simulink model "attitude_cbf"  (R2020b)
settings: Solver=VariableStepAuto  StartTime=0.0  StopTime=10.0  RelTol=1e-3
settings Model: Creator=kt012  LastModifiedBy=kt012

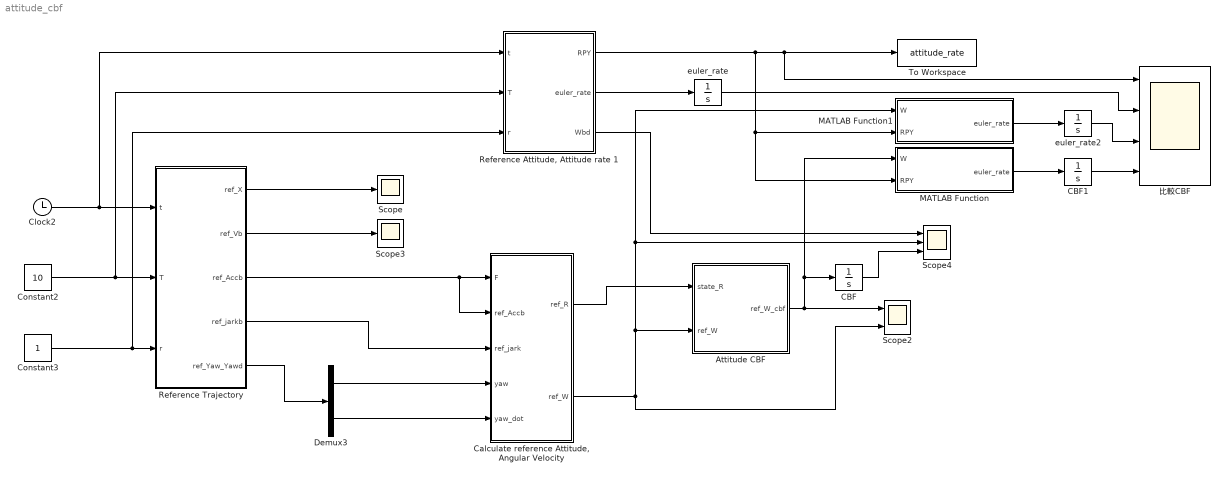
== system attitude_cbf ==
  Attitude CBF : MATLAB Function  TreatAsAtomicUnit=on
  CBF : Integrator  InitialCondition=[0.0403 0 0];
  CBF1 : Integrator  InitialCondition=[0.0403 0 0];
  "Calculate reference Attitude, Angular Velocity" : MATLAB Function  TreatAsAtomicUnit=on
  Clock2 : Clock
  Constant2 : Constant  Value=10
  Constant3 : Constant
  Demux3 : Demux  Outputs=2
  MATLAB Function : MATLAB Function  TreatAsAtomicUnit=on
  MATLAB Function1 : MATLAB Function  TreatAsAtomicUnit=on
  "Reference Attitude, Attitude rate 1" : MATLAB Function  TreatAsAtomicUnit=on
  Reference Trajectory : MATLAB Function  TreatAsAtomicUnit=on
  Scope : Scope
  Scope2 : Scope  NumInputPorts=2
  Scope3 : Scope
  Scope4 : Scope  NumInputPorts=3
  To Workspace : ToWorkspace  VariableName=attitude_rate  SaveFormat=Structure  SampleTime=-1
  euler_rate : Integrator  InitialCondition=[0.0403 0 0];
  euler_rate2 : Integrator  InitialCondition=[0.0403 0 0];
  比較CBF : Scope  NumInputPorts=4
  wires:
  Clock2/1 -> "Reference Attitude, Attitude rate 1"/1(t), Reference Trajectory/1(t)
  Constant3/1 -> "Reference Attitude, Attitude rate 1"/3(r), Reference Trajectory/3(r)
  Constant2/1 -> "Reference Attitude, Attitude rate 1"/2(T), Reference Trajectory/2(T)
  Reference Trajectory/1(ref_X) -> Scope/1
  Reference Trajectory/2(ref_Vb) -> Scope3/1
  Reference Trajectory/3(ref_Accb) -> "Calculate reference Attitude, Angular Velocity"/2(ref_Accb), "Calculate reference Attitude, Angular Velocity"/1(F)
  Reference Trajectory/4(ref_jarkb) -> "Calculate reference Attitude, Angular Velocity"/3(ref_jark)
  Reference Trajectory/5(ref_Yaw_Yawd) -> Demux3/1
  Demux3/1 -> "Calculate reference Attitude, Angular Velocity"/4(yaw)
  Demux3/2 -> "Calculate reference Attitude, Angular Velocity"/5(yaw_dot)
  "Calculate reference Attitude, Angular Velocity"/1(ref_R) -> Attitude CBF/1(state_R)
  "Calculate reference Attitude, Angular Velocity"/2(ref_W) -> Scope2/2, MATLAB Function1/1(W), Scope4/2, Attitude CBF/2(ref_W)
  Attitude CBF/1(ref_W_cbf) -> Scope2/1, MATLAB Function/1(W), CBF/1
  "Reference Attitude, Attitude rate 1"/3(Wbd) -> Scope4/1
  "Reference Attitude, Attitude rate 1"/1(RPY) -> MATLAB Function/2(RPY), MATLAB Function1/2(RPY), 比較CBF/1, To Workspace/1
  CBF/1 -> Scope4/3
  "Reference Attitude, Attitude rate 1"/2(euler_rate) -> euler_rate/1
  euler_rate/1 -> 比較CBF/2
  euler_rate2/1 -> 比較CBF/3
  MATLAB Function/1(euler_rate) -> CBF1/1
  MATLAB Function1/1(euler_rate) -> euler_rate2/1
  CBF1/1 -> 比較CBF/4

== matlab function attitude_cbf/Reference Attitude, Attitude rate 1 ==
  data: RPY output; euler_rate output; Wbd output; t input; T input; r input
function [RPY, euler_rate, Wbd] = fcn(t,T,r)
% 軌道生成
w = 2 * pi/T;          % 角周波数

% 中心　半径　　
c = [0;0;0];

% Flat Outputから内部状態と入力揚力を計算
% 各軸の単位行列
e1 = [1; 0; 0];e2 = [0; 1; 0];e3 = [0; 0; 1];
% ドローンの質量　重力加速度
mQ = 0.027; g = 9.8;


x = c + r*[sin(w*t); cos(w*t); 0];         % 位置の軌道の位置
dx = r*[w*cos(w*t); -w*sin(w*t); 0];       % 速度の軌道
d2x = r*[-w^2*sin(w*t); -w^2*cos(w*t); 0]; % 加速度の軌道
d3x = r*[-w^3*cos(w*t); w^3*sin(w*t); 0];  % 加加速度の軌道
d4x = r*[w^4*sin(w*t); w^4*cos(w*t); 0];   % 加加加速度の軌道

alpha = 0;                                 
d_alpha = 0;                               
d2x(3) = d2x(3)+g;

pitch = atan( ( d2x(1)*cos(alpha) + d2x(2)*sin(alpha) ) / (d2x(3)));                                                        
roll = atan( ( d2x(1)*sin(alpha) - d2x(2)*cos(alpha) ) / sqrt( (d2x(3))^2 + ( d2x(1)*cos(alpha) + d2x(2)*sin(alpha) )^2));

rollS = sin(roll); rollC = cos(roll);           
pitchS = sin(pitch); pitchC = cos(pitch);       
yawS = sin(alpha); yawC = cos(alpha);           


% desired Roll rate
roll_rate_bunshi = d2x(3)^2 * ( d3x(1)*yawS - d3x(2)*yawC + d_alpha * (d2x(1)*yawC + d2x(2)*yawS) ) - d2x(3)*d3x(3)*(d2x(1)*yawS - d2x(2)*yawC) + (d2x(1)*yawC + d2x(2)*yawS)*(d_alpha*(d2x(1)^2 + d2x(2)^2) - d2x(1)*d3x(2) + d2x(2)*d3x(1));
roll_rate_bunbo = (d2x(1)^2 + d2x(2)^2 + d2x(3)^2) * sqrt(d2x(3)^2 + ( d2x(1)*yawC + d2x(2)*yawS )^2);
roll_rate = roll_rate_bunshi / roll_rate_bunbo;

% desired Pitch rate
pitch_rate_bunshi = d2x(3)*(d3x(1)*yawC + d3x(2)*yawS) - d3x(3)*(d2x(1)*yawC + d2x(2)*yawS) - d2x(3)*d_alpha*(d2x(1)*yawS + d2x(2)*yawC);
pitch_rate_bunbo = d2x(3)^2 + ( d2x(1)*yawC + d2x(2)*yawS )^2;
pitch_rate = pitch_rate_bunshi / pitch_rate_bunbo;

W = [1 0      -pitchS;
     0 rollC  pitchC * rollS;
     0 -rollS pitchC * rollC] * [roll_rate;pitch_rate;d_alpha];

RPY = [roll, pitch, alpha]';
euler_rate = [roll_rate;pitch_rate;d_alpha];
Wbd = W;

== matlab function attitude_cbf/Calculate reference Attitude, Angular Velocity ==
  data: ref_R output; ref_W output; F input; ref_Accb input; ref_jark input; yaw input; yaw_dot input
function [ref_R,ref_W]= fcn(F, ref_Accb, ref_jark, yaw, yaw_dot)

% Flat Outputから内部状態と入力揚力を計算

m = 0.03;
F = F;
Xc = [cos(yaw) sin(yaw) 0]';          % よー角のベクトル　Rc(3)
Yc = [-sin(yaw) cos(yaw) 0]';
dXc = yaw_dot * Yc; % よー角のベクトルの微分
dYc = -yaw_dot * Xc; 

% 所望の姿勢を計算している
% 軌道の加速度のベクトル: b3 を計算
Zb = F / norm(F);   
%
Xb = cross(Yc, Zb)/norm(cross(Yc, Zb));
Yb = cross(Zb, Xb);
ref_R = [Xb Yb Zb] ;

% 加加速度ベクトルを計算
dfZb = ref_jark;
  
% 目標の姿勢のz軸方向のベクトルの微分を計算
dZb = dfZb/norm(F) - F * dot(F, dfZb)/norm(F)^3; % Zb_dot---------- dot(　fb1/norm(fb1) )

% 目標の姿勢のx軸方向のベクトルを計算
dnorm_Zb_Xc2 = norm(cross(dYc, Zb) + cross(Yc, dZb));
dXb = (cross(dYc, Zb) + cross(Yc, dZb))/dnorm_Zb_Xc2 - cross(Yc, Zb) * dot(cross(Yc, Zb),( cross(dYc, Zb) + cross(Yc, dZb)))/dnorm_Zb_Xc2^3;
   
% 目標の姿勢のy軸方向のベクトルを計算
dYb = cross(dZb, Xb) + cross(Zb, dXb) ;  %dot_b2 = dotb3とb1 の外積と　b3とdot_b1の外積　の和　--------- dot(cross(b3, b1))


wy = dot(Xb, ref_jark) / dot(Zb, ref_Accb);
wx = - dot(Yb, ref_jark) / dot(Zb, ref_Accb);
wz = (yaw_dot * dot(Xc, Xb) + wy * dot(Yc, Zb))/norm(cross(Yc, Zb));
ref_W = [wx wy wz];

== matlab function attitude_cbf/MATLAB Function ==
  data: W input; euler_rate output; RPY input
function euler_rate = fcn(W, RPY)
roll = RPY(1);
pitch = RPY(2);
yaw = RPY(3);
rollS = sin(roll); rollC = cos(roll);           
pitchS = sin(pitch); pitchC = cos(pitch);       


euler_rate = pinv([1 0 -pitchS;
     0 rollC  pitchC * rollS;
     0 -rollS pitchC * rollC]) * W;

== matlab function attitude_cbf/MATLAB Function1 ==
  data: W input; euler_rate output; RPY input
function euler_rate = fcn(W, RPY)
roll = RPY(1);
pitch = RPY(2);
yaw = RPY(3);
rollS = sin(roll); rollC = cos(roll);           
pitchS = sin(pitch); pitchC = cos(pitch);       


euler_rate = pinv([1 0 -pitchS;
     0 rollC  pitchC * rollS;
     0 -rollS pitchC * rollC]) * W';

== matlab function attitude_cbf/Attitude CBF ==
  data: state_R input; ref_W input; ref_W_cbf output
function ref_W_cbf = fcn(state_R, ref_W)

theta = 1;
coder.extrinsic('quadprog')
ref_W_cbf = zeros(3, 1);
e3 = [0; 0; 1];
e3_wedge = [0 -1 0; 1 0 0; 0 0 0];
H = eye(3);
f = -ref_W;

A = e3'*state_R*e3_wedge;
B = ( e3'*state_R*e3 - cos(theta) );

tmp  = quadprog(H, f, A, B);
ref_W_cbf = [tmp(1) tmp(2) tmp(3)];

== matlab function attitude_cbf/Reference Trajectory ==
  data: ref_X output; ref_Vb output; ref_Accb output; ref_jarkb output; t input; T input; r input; ref_Yaw_Yawd output
function [ref_X, ref_Vb, ref_Accb, ref_jarkb, ref_Yaw_Yawd] = fcn(t,T,r)
% 軌道生成
w = 2 * pi/T;          % 角周波数

% 中心　半径　　
c = [0;0;0];

ref_X = c + r*[sin(w*t); cos(w*t); 0];
ref_Vb = r*[w*cos(w*t); -w*sin(w*t); 0];
ref_Accb = [-r*w^2*sin(w*t); -r*w^2*cos(w*t); 9.8];
ref_jarkb = r*[-w^3*cos(w*t); w^3*sin(w*t); 0];
ref_Yaw_Yawd = [0, 0]';
